simulink model "SWC_ETE_type"  (R2024a)
settings: Solver=FixedStepDiscrete  StartTime=0.0  StopTime=10.0  RelTol=1e-3
values from neighbouring files (symbols this model uses):
  C_FOC_SAMPLE_TIME = single(0.0001)    [vcu_local_hdr.m]
  ENUM_SENSORFOCMODE_CURRENTRDCTEMP = uint8(  2  )    [vcu_local_hdr.m]
  ENUM_SENSORFOCMODE_FAKERDC = uint8(  1  )    [vcu_local_hdr.m]
  ENUM_SENSORFOCMODE_RDCALIGN = uint8(  3  )    [vcu_local_hdr.m]
  ENUM_SENSORMODE_RDC = uint8(  0  )    [vcu_local_hdr.m]
  FALSE = boolean( 0 )    [vcu_local_hdr.m]
  MINUSONE_PI = single( -pi)    [vcu_local_hdr.m]
  PI = single( pi )    [vcu_local_hdr.m]
  SPD_GAIN = single(2*pi/60)    [vcu_local_hdr.m]
  TRUE = boolean( 1 )    [vcu_local_hdr.m]
  TWO_PI = single( 2*pi)    [vcu_local_hdr.m]
  ZERO_FLOAT = single(0)    [vcu_local_hdr.m]
undefined symbols (not defined in the file or in its folder): KFOC_25Amb_degC, KFOC_ADCReadEnum_enum, KFOC_DCBusLPF_c, KFOC_DCBusUseRaw_flg, KFOC_DCBusVoltage_V_ovrdflg, KFOC_DCBusVoltage_V_ovrdval, KFOC_FltActn_flg_ovrdflg, KFOC_FltActn_flg_ovrdfval, KFOC_GateICDisable_flg, KFOC_GateICEnable_flg, KFOC_GateICTempConst_raw, KFOC_IdCmd_A_ovrdflg, KFOC_IdCmd_A_ovrdfval, KFOC_IqCmd_A_ovrdflg, KFOC_IqCmd_A_ovrdfval, KFOC_OpMod_enum, KFOC_OpMod_enum_ovrdflg, KFOC_OpMod_enum_ovrdval, KFOC_PosnOffset_flg_ovrdflg, KFOC_PosnOffset_rad_ovrdval, KFOC_PWMidle_flg, KFOC_RotPosnOffset_rad_ovrdflg, KFOC_RotPosnOffset_rad_ovrdval, KFOC_SensorMode_enum, KFOC_SpdCmd_RPM, KFOC_TCTS_const, KFOC_VdCmd_V, KFOC_VqCmd_V, KFOC_VTS25_V
libraries: simulink x6, rot x2, GRC_Lib x1, pcs_grc x1, rot_grc x1, hdlsllib x1, CCM_FVT x1, dgh_grc x1, pdc_grc x1
(part 1 of 2)
settings Model: DataDictionary=APPTypes.sldd  Creator=FVT22063  LastModifiedBy=FVT22063
settings DataIOCC: SaveFormat=StructureWithTime
settings OptimizationCC: DefaultParameterBehavior=Inlined  EnhancedBackFolding=on  PassReuseOutputArgsAs=Individual arguments  ZeroExternalMemoryAtStartup=off  ZeroInternalMemoryAtStartup=off  OptimizeBlockOrder=speed  DifferentSizesBufferReuse=on  OptimizationCustomize=off  EfficientTunableParamExpr=on
settings DebuggingCC: ParameterTunabilityLossMsg=error
settings HardwareCC: ProdBitPerPointer=32  ProdBitPerSizeT=32  ProdBitPerPtrDiffT=32  ProdLargestAtomicInteger=Long  ProdLargestAtomicFloat=Double  ProdWordSize=32  ProdLongLongMode=on  ProdHWDeviceType=ARM Compatible->ARM Cortex-M
settings ModelReferenceCC: ModelReferenceNumInstancesAllowed=Single
settings SFSimCC: SimCustomHeaderCode="#include \"FVTMC_API.h\""  SimUserSources=FVTMC_API.c  MATLABDynamicMemAlloc=off
settings RTWCC: Description=AUTOSAR  SystemTargetFile=autosar.tlc  GenCodeOnly=on  TemplateMakefile=ert_default_tmf  PortableWordSizes=on
settings CodeAppCC: ForceParamTrailComments=on  IgnoreCustomStorageClasses=off  OperatorAnnotations=on  SimulinkDataObjDesc=on  SFDataObjDesc=on  InsertBlockDesc=on
settings STFCustomTargetCC: UtilityFuncGeneration=Shared location  MultiwordLength=256  ParMdlRefBuildCompliant=on  CompOptLevelCompliant=on  IncludeMdlTerminateFcn=off  CombineOutputUpdateFcns=on  SuppressErrorStatus=on  ERTCustomFileBanners=on  SupportNonFinite=off  SupportComplex=off  SupportContinuousTime=off  SupportNonInlinedSFcns=off  RemoveResetFunc=on  MATLABClassNameForMDSCustomization=Simulink.SoftwareTarget.ERTCustomization  AutosarCompliant=on  GRTInterface=off  GenerateSharedConstants=off  LookupTableObjectStructAxisOrder=2,1,3,4,...  LUTObjectStructOrderEvenSpacing=Size,Table,Breakpoints  SystemTargetFile=autosar.tlc
settings ERTTargetCC: TargetLangStandard=C99 (ISO)  UtilityFuncGeneration=Shared location  ConcurrentExecutionCompliant=off  IncludeMdlTerminateFcn=off  SuppressErrorStatus=on  SupportNonFinite=off  SupportComplex=off  ModelStepFunctionPrototypeControlCompliant=off  CPPClassGenCompliant=off  AutosarCompliant=on  GenerateSharedConstants=off  LookupTableObjectStructAxisOrder=2,1,3,4,...  LUTObjectStructOrderEvenSpacing=Size,Table,Breakpoints  GenerateASAP2=on  InlinedParameterPlacement=NonHierarchical  ERTCustomFileTemplate=example_file_process.tlc  ConvertIfToSwitch=off  SuppressUnreachableDefaultCases=off  BooleanTrueId=true_MatlabRTW  BooleanFalseId=false_MatlabRTW

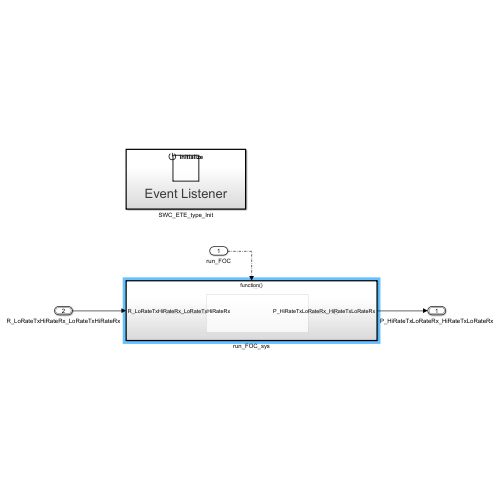
[thumbnail: Simulink's stored preview of the top-level diagram]
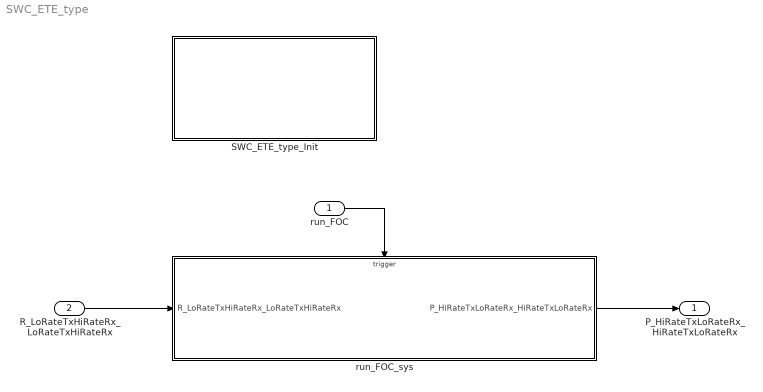
== system SWC_ETE_type ==
  run_FOC : Inport  OutputFunctionCall=on
  R_LoRateTxHiRateRx_LoRateTxHiRateRx : Inport  Port=2  OutDataTypeStr=Bus: DT_LoRateTxHiRateRx  PortDimensions=1  BusOutputAsStruct=on
  SWC_ETE_type_Init : Subsystem
  run_FOC_sys : Subsystem
  P_HiRateTxLoRateRx_HiRateTxLoRateRx : Outport  OutDataTypeStr=Bus: DT_HiRateTxLoRateRx  PortDimensions=1  BusOutputAsStruct=on
  wires:
  R_LoRateTxHiRateRx_LoRateTxHiRateRx/1 -> run_FOC_sys/1(R_LoRateTxHiRateRx_LoRateTxHiRateRx)
  run_FOC_sys/1(P_HiRateTxLoRateRx_HiRateTxLoRateRx) -> P_HiRateTxLoRateRx_HiRateTxLoRateRx/1
  run_FOC/1 -> run_FOC_sys/Trigger

== system SWC_ETE_type/SWC_ETE_type_Init ==
  Event Listener : EventListener  EventName=reset

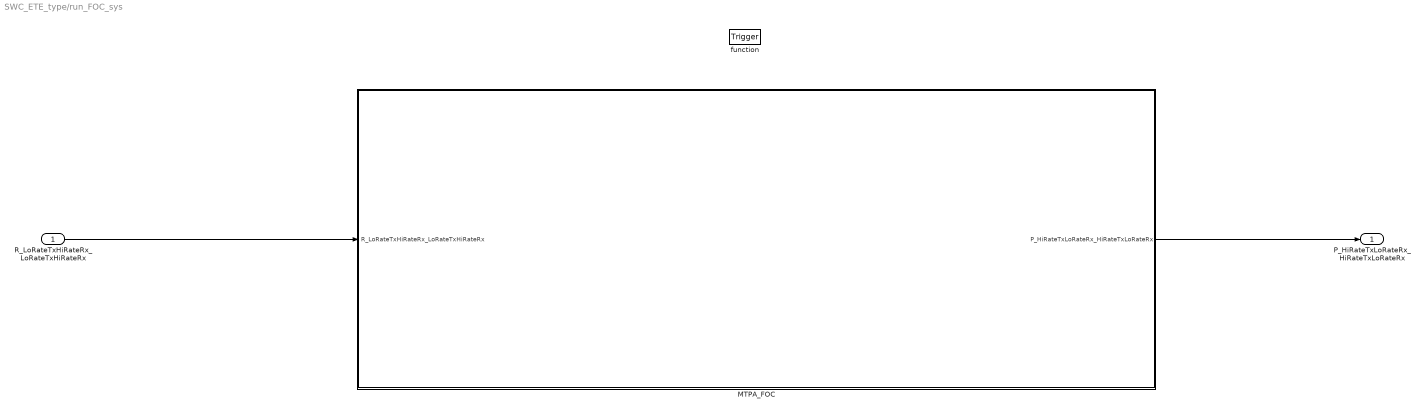
== system SWC_ETE_type/run_FOC_sys ==
  R_LoRateTxHiRateRx_LoRateTxHiRateRx : Inport
  function : TriggerPort  TriggerType=function-call  VariantControl=(inherit)
  MTPA_FOC : Subsystem  TreatAsAtomicUnit=on
      settings: RTWSystemCode=Nonreusable function  RTWFcnNameOpts=Use subsystem name  RTWFileNameOpts=Use subsystem name
  P_HiRateTxLoRateRx_HiRateTxLoRateRx : Outport
  wires:
  R_LoRateTxHiRateRx_LoRateTxHiRateRx/1 -> MTPA_FOC/1(R_LoRateTxHiRateRx_LoRateTxHiRateRx)
  MTPA_FOC/1(P_HiRateTxLoRateRx_HiRateTxLoRateRx) -> P_HiRateTxLoRateRx_HiRateTxLoRateRx/1

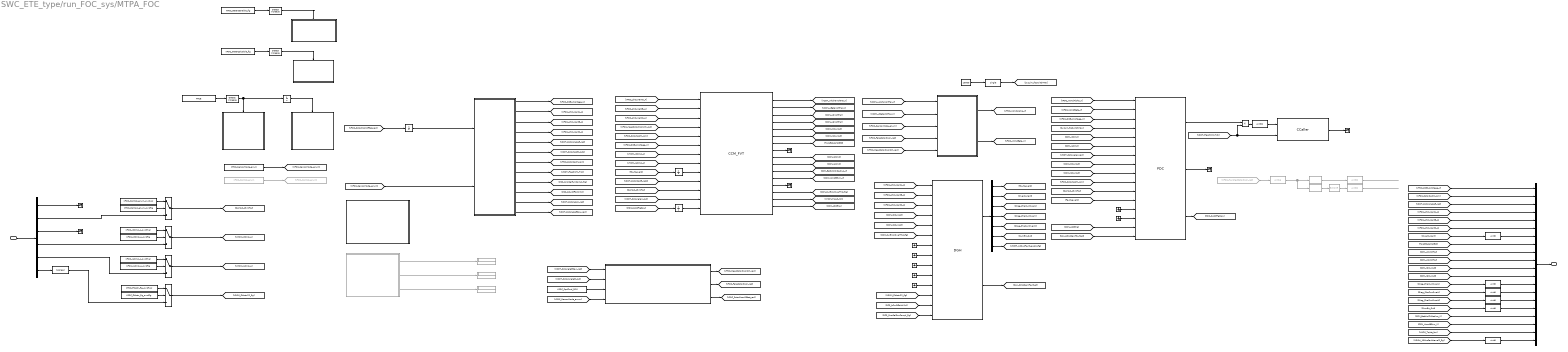
== system SWC_ETE_type/run_FOC_sys/MTPA_FOC ==
  R_LoRateTxHiRateRx_LoRateTxHiRateRx : Inport
  ADC_RDC_Read : Subsystem  TreatAsAtomicUnit=on
      settings: RTWSystemCode=Nonreusable function  RTWFcnNameOpts=Use subsystem name  RTWFileNameOpts=Use subsystem name
  Bit Shift : hdlsllib/Logic and Bit Operations/Bit Shift  Commented=on  mode=Shift Right Logical  N=8
  Bitwise Operator : simulink/Logic and Bit Operations/Bitwise Operator  Commented=on  logicop=AND  UseBitMask=on  BitMask=0xFF00  BitMaskRealWorld=Stored Integer
  Bitwise Operator1 : simulink/Logic and Bit Operations/Bitwise Operator  Commented=on  logicop=AND  UseBitMask=on  BitMask=0x00FF  BitMaskRealWorld=Stored Integer
  Bus Creator : BusCreator  Inputs=20  OutDataTypeStr=Bus: DT_HiRateTxLoRateRx  NonVirtualBus=on
  Bus Selector : BusSelector  OutputSignals=VDGH_FaultLevel2_flg,OverCurrent,Diag_bPhaCurrOverU,Diag_bPhaCurrOverV,Diag_bPhaCurrOverW,SumErr_Out,VDGH_100usFaultLevel2_flg
  Bus Selector1 : BusSelector  OutputSignals=u8_OpMod_stMotAct,u8_OpMod_stIvtrTar,f32_SysLim_frqSwitchMax,f32_VMCM_IdCmd_A,f32_VMCM_IqCmd_A,u8_VDSM_FltActn22_flg
  C Caller1 : CCaller  FunctionName=pwm_set_duty  PortSpecificationStruct="%)30     .      0   8    (     @         %    \"     (    !     0         %  0 \"0    $    _    07)G3F%M90  4&]R=$YA;64 4V-O<&4     26YD97@     5'EP90      4VEZ90      27-';&]B86P   X   !     !@    @    $          4    (     0    X    !         !     .    =3,R07)R87DS7U1I8VL   X   !     !@    @    $          4    (     0    X    !         !     .    =3,R07)R87DS7U1I8VL   X   !     !@    @    $          4    (     0    L    !         !     +    26YP=71/=71P=70       X    X    !@    @    &          4    (     0    $    !          D    (               .    .     8    (    !          %    \"     $    &     0         0    !@   '5I;G0S,@  #@   #     &    \"     0         !0    @    !     0    $         $  ! #,    .    ,     8    (    \"0(        %    \"     $    !     0         \"  $       X   !     !@    @    $          4    (     0    L    !         !     +    <&5R:6]D7U1I8VL       X   !     !@    @    $          4    (     0    L    !         !     +    <&5R:6]D7U1I8VL       X    X    !@    @    $          4    (     0    4    !         !     %    26YP=70    .    .     8    (    !@         %    \"     $    !     0         )    \"            / _#@   #@    &    \"     0         !0    @    !    !@    $         $     8   !U:6YT,S(   X    P    !@    @    $          4    (     0    $    !         !   0 Q    #@   #     &    \"     D\"        !0    @    !     0    $          @ !"
  CCM_FVT : CCM_FVT/CCM_FVT  SystemSampleTime=-1  VariantActivationTime=update diagram  AllowFlexibleInterface=on  Latency=0  AutoFrameSizeCalculation=off
  Cast To Boolean : DataTypeConversion  OutDataTypeStr=boolean  SaturateOnIntegerOverflow=off  RndMeth=Floor
  Constant : Constant  Value=10000
  Constant1 : Constant  Value=KFOC_GateICDisable_flg
  Constant10 : Constant  Value=KFOC_OpMod_enum_ovrdflg
  Constant11 : Constant  Value=KFOC_OpMod_enum_ovrdval
  Constant12 : Constant  Value=KFOC_FltActn_flg_ovrdflg
  Constant13 : Constant  Value=KFOC_SensorMode_enum
  Constant14 : Constant  Value=KFOC_FltActn_flg_ovrdfval
  Constant2 : Constant  Value=KFOC_SpdCmd_RPM
  Constant3 : Constant  Value=KFOC_GateICEnable_flg
  Constant4 : Constant  Commented=on  Value=KFOC_OpMod_enum
  Constant5 : Constant  Value=KFOC_IdCmd_A_ovrdflg
  Constant6 : Constant  Value=KFOC_IdCmd_A_ovrdfval
  Constant7 : Constant  Value=TRUE
  Constant8 : Constant  Value=KFOC_IqCmd_A_ovrdflg
  Constant9 : Constant  Value=KFOC_IqCmd_A_ovrdfval
  DGH : dgh_grc/DGH  SystemSampleTime=-1  VariantActivationTime=update diagram  AllowFlexibleInterface=on  Latency=0  AutoFrameSizeCalculation=off
  Data Type Conversion : DataTypeConversion  OutDataTypeStr=single  SaturateOnIntegerOverflow=off  RndMeth=Floor
  Data Type Conversion1 : DataTypeConversion  OutDataTypeStr=uint32  SaturateOnIntegerOverflow=off  RndMeth=Floor
  Data Type Conversion{2..5,9..10} (6 alike) : DataTypeConversion  OutDataTypeStr=uint8  SaturateOnIntegerOverflow=off  RndMeth=Floor
  Data Type Conversion6 : DataTypeConversion  Commented=on  OutDataTypeStr=uint32  SaturateOnIntegerOverflow=off  RndMeth=Floor
  Data Type Conversion7 : DataTypeConversion  Commented=on  OutDataTypeStr=uint32  SaturateOnIntegerOverflow=off  RndMeth=Floor
  Data Type Conversion8 : DataTypeConversion  Commented=on  OutDataTypeStr=uint16  SaturateOnIntegerOverflow=off  RndMeth=Floor
  Detect Increase : simulink/Logic and Bit Operations/Detect Increase  vinit=0.0  OutDataTypeStr=boolean
  Detect Increase1 : simulink/Logic and Bit Operations/Detect Increase  vinit=0.0  OutDataTypeStr=boolean
  Detect Increase2 : simulink/Logic and Bit Operations/Detect Increase  vinit=0.0  OutDataTypeStr=boolean
  Disable_GateIC : Subsystem
  Display : Display  Commented=on
  Display1 : Display  Commented=on
  Display2 : Display  Commented=on
  Enable_GateIC : Subsystem
  FOC_Mode_Judge : Subsystem  TreatAsAtomicUnit=on
      settings: RTWSystemCode=Nonreusable function  RTWFcnNameOpts=Use subsystem name  RTWFileNameOpts=Use subsystem name
  From42 : From  Commented=on  GotoTag=VFOC_HandledRotorPosn_rad
  GateDirver_Temp_Read : Subsystem  Commented=on  TreatAsAtomicUnit=on
      settings: RTWSystemCode=Nonreusable function  RTWFcnNameOpts=Use subsystem name  RTWFileNameOpts=Use subsystem name
  Goto24 : Goto  Commented=on  GotoTag=VFOC_OpMod_enum
  Ground{,1..6} (7 alike) : Ground
  PDC : pdc_grc/PDC  SystemSampleTime=-1  VariantActivationTime=update diagram  AllowFlexibleInterface=on  Latency=0  AutoFrameSizeCalculation=off
  PWM_idle_Mode : Subsystem
  Product : Product
  RotorPositionHandle : Subsystem
  Subsystem : Subsystem
  Subsystem1 : Subsystem
  Switch{,1..3} (4 alike) : Switch  Criteria=u2 ~= 0  SaturateOnIntegerOverflow=off  InputSameDT=off
  Terminator{,1..5} (6 alike) : Terminator
  Unit Delay{,1..3} (4 alike) : UnitDelay  SampleTime=-1  HasFrameUpgradeWarning=on
  P_HiRateTxLoRateRx_HiRateTxLoRateRx : Outport
  wires:
  Detect Increase/1 -> Unit Delay/1, Subsystem/Enable
  ADC_RDC_Read/1(VFOC_DCBusVoltage_V) -> [VFOC_DCBusVoltage_V]
  Data Type Conversion6/1 -> ?  "RotorPosn_100rad_LowByte"
  [VFOC_SensorMode_enum] -> RotorPositionHandle/4(VFOC_SensorMode_enum)
  RotorPositionHandle/1(VFOC_MeasRotorPosn2Pi_rad) -> [VFOC_MeasRotorPosn2Pi_rad]
  [VCCM_uBetaVoltTar_V] -> FOC_Mode_Judge/2(VCCM_uBetaVoltTar_V)
  Data Type Conversion8/1 -> Bitwise Operator/1, Bitwise Operator1/1
  Constant7/1 -> Detect Increase/1
  ADC_RDC_Read/4(VFOC_phCurrentC_A) -> [VFOC_phCurrentC_A]
  GateDirver_Temp_Read/1(Out1) -> Display/1
  [VFOC_SensorMode_enum] -> FOC_Mode_Judge/3(VFOC_SensorMode_enum)
  Data Type Conversion7/1 -> ?  "RotorPosn_100rad_HighByte"
  [VFOC_MeasRotorPosn2Pi_rad] -> FOC_Mode_Judge/5(VFOC_MeasRotorPosn2Pi_rad)
  [VFOC_FakeRotorPosn_rad] -> FOC_Mode_Judge/4(VFOC_FakeRotorPosn_rad)
  Bit Shift/1 -> Data Type Conversion7/1
  RotorPositionHandle/2(VFOC_FakeRotorPosn_rad) -> [VFOC_FakeRotorPosn_rad]
  Bitwise Operator/1 -> Bit Shift/1
  GateDirver_Temp_Read/2(Out2) -> Display1/1
  ADC_RDC_Read/3(VFOC_phCurrentB_A) -> [VFOC_phCurrentB_A]
  [VFOC_MeasRotorPosn2Pi_rad] -> CCM_FVT/4
  Constant13/1 -> [VFOC_SensorMode_enum]
  GateDirver_Temp_Read/3(Out3) -> Display2/1
  Bitwise Operator1/1 -> Data Type Conversion6/1
  Constant2/1 -> RotorPositionHandle/3(VFOC_SpdCmd_rpm)
  [VCCM_uAlphaVoltTar_V] -> FOC_Mode_Judge/1(VCCM_uAlphaVoltTar_V)
  [VFOC_DCBusVoltage_V] -> CCM_FVT/6
  [VFOC_RotorSpdM_rpm] -> CCM_FVT/5
  ADC_RDC_Read/5(VROT_RotorAngleE_rad) -> [VROT_RotorAngleE_rad]
  [VROT_RotorAngleE_rad] -> RotorPositionHandle/2(VROT_RotorAngleE_rad)
  ADC_RDC_Read/6(VROT_RotorSpdE_rads) -> [VROT_RotorSpdE_rads]
  ADC_RDC_Read/7(VROT_RotorSpdM_rpm) -> [VFOC_RotorSpdM_rpm]
  Unit Delay/1 -> Subsystem1/Enable
  Detect Increase1/1 -> Disable_GateIC/Enable
  Detect Increase2/1 -> Enable_GateIC/Enable
  Constant1/1 -> Detect Increase1/1
  Constant3/1 -> Detect Increase2/1
  FOC_Mode_Judge/1(VFOC_VcmdAlpha_V) -> [VFOC_VcmdAlpha_V]
  FOC_Mode_Judge/2(VFOC_VcmdBeta_V) -> [VFOC_VcmdBeta_V]
  [VFOC_DCBusVoltage_V] -> PDC/3
  [VFOC_RotorSpdM_rpm] -> PDC/10
  ADC_RDC_Read/2(VFOC_phCurrentA_A) -> [VFOC_phCurrentA_A]
  [VFOC_phCurrentA_A] -> CCM_FVT/1
  [VFOC_phCurrentB_A] -> CCM_FVT/2
  [VFOC_phCurrentC_A] -> CCM_FVT/3
  CCM_FVT/1 -> [VCCM_uAlphaVoltTar_V]
  CCM_FVT/2 -> [VCCM_uBetaVoltTar_V]
  CCM_FVT/3 -> [CCM_uDVoltTar]
  CCM_FVT/4 -> [CCM_uQVoltTar]
  [VFOC_VcmdAlpha_V] -> PDC/1
  [VFOC_VcmdBeta_V] -> PDC/2
  [SysLim_frqSwitchMax] -> PDC/4
  Constant/1 -> Data Type Conversion/1
  Data Type Conversion/1 -> [SysLim_frqSwitchMax]
  CCM_FVT/5 -> [CCM_iDCurrAct]
  CCM_FVT/6 -> [CCM_iQCurrAct]
  CCM_FVT/9 -> [CCM_idCmd]
  CCM_FVT/10 -> [CCM_iqCmd]
  [CCM_idCmd] -> PDC/5
  [CCM_iqCmd] -> PDC/6
  [CCM_iDCurrAct] -> PDC/8
  [CCM_iQCurrAct] -> PDC/9
  [VROT_RotorSpdE_rads] -> CCM_FVT/10
  [OpMod_stlvtrTar] -> PDC/11
  [OpMod_stlvtrTar] -> CCM_FVT/11
  Constant4/1 -> Goto24/1
  PDC/1 -> Product/1  "PDC_Ivtr1ModCmd"
  C Caller1/1 -> Terminator/1
  ADC_RDC_Read/8(VROT_FreqPWM_Tick) -> [VROT_FreqPWM_Tick]
  [VROT_FreqPWM_Tick] -> Product/2, C Caller1/2
  CCM_FVT/16 -> [CCM_ASCEna]
  [CCM_ASCEna] -> PDC/15
  Product/1 -> Data Type Conversion1/1
  Data Type Conversion1/1 -> C Caller1/1
  ADC_RDC_Read/11(VROT_RotAngleV_rad) -> [VROT_RotAngleV_rad]
  [VROT_RotAngleV_rad] -> CCM_FVT/12
  [VROT_RotAngleV_rad] -> PDC/7
  PDC/3 -> [PDC_bASCFlgRaw]
  Unit Delay1/1 -> CCM_FVT/13
  [PDC_bASCFlgRaw] -> Unit Delay1/1
  RotorPositionHandle/3(VFOC_RotorPosnOffset_rad) -> [VFOC_RotorPosnOffset_rad]
  [VFOC_RotorPosnOffset_rad] -> Unit Delay2/1
  Unit Delay2/1 -> ADC_RDC_Read/1(VFOC_RotPosnOfstDelay_rad)  "VFOC_RotPosnOfstDelay_rad"
  [CCM_iDCurrAct] -> DGH/4
  [CCM_iQCurrAct] -> DGH/5
  [VFOC_phCurrentA_A] -> DGH/1
  [VFOC_phCurrentC_A] -> DGH/3
  [VFOC_phCurrentB_A] -> DGH/2
  CCM_FVT/14 -> [CCM_CurErrorOverThd_flg]
  [CCM_CurErrorOverThd_flg] -> DGH/6
  [PCS_bCurOffsVolVld] -> DGH/13
  [PCS_SnsrSelfLrnCompl_flg] -> DGH/14
  ADC_RDC_Read/10(PCS_bCurOffsVolVld_flg) -> [PCS_bCurOffsVolVld]
  ADC_RDC_Read/9(PCS_SnsrSelfLrnCompl_flg) -> [PCS_SnsrSelfLrnCompl_flg]
  Unit Delay3/1 -> CCM_FVT/9
  [FaultLevel2] -> Unit Delay3/1
  DGH/2 -> [bsw_bPosSenrFaultLat]
  [bsw_bPosSenrFaultLat] -> PDC/16
  [FaultLevel2] -> PDC/12
  From42/1 -> Data Type Conversion8/1
  DGH/1 -> Bus Selector/1
  Bus Selector/1 -> [FaultLevel2]  "<VDGH_FaultLevel2_flg>"
  R_LoRateTxHiRateRx_LoRateTxHiRateRx/1 -> Bus Selector1/1
  Bus Selector1/1 -> Terminator2/1  "<u8_OpMod_stMotAct>"
  Bus Selector1/2 -> Switch2/3  "<u8_OpMod_stIvtrTar>"
  Bus Selector1/3 -> Terminator1/1  "<f32_SysLim_frqSwitchMax>"
  [VMCM_IdCmd_A] -> CCM_FVT/7
  [VMCM_IqCmd_A] -> CCM_FVT/8
  Bus Selector1/5 -> Switch1/3  "<f32_VMCM_IqCmd_A>"
  [VDSM_FltActn22_flg] -> DGH/12
  Bus Selector1/6 -> Cast To Boolean/1  "<u8_VDSM_FltActn22_flg>"
  Bus Creator/1 -> P_HiRateTxLoRateRx_HiRateTxLoRateRx/1
  [VFOC_DCBusVoltage_V] -> Bus Creator/1
  [VFOC_RotorSpdM_rpm] -> Bus Creator/2
  [VROT_RotorAngleE_rad] -> Bus Creator/3
  [VFOC_phCurrentB_A] -> Bus Creator/5
  [VFOC_phCurrentC_A] -> Bus Creator/6
  [VFOC_phCurrentA_A] -> Bus Creator/4
  Bus Selector/2 -> [OverCurrent]  "<OverCurrent>"
  [OverCurrent] -> Data Type Conversion2/1
  CCM_FVT/7 -> [TorqEst_tqMotEst]
  [TorqEst_tqMotEst] -> Bus Creator/8
  [CCM_uQVoltTar] -> Bus Creator/10
  [CCM_uDVoltTar] -> Bus Creator/9
  [CCM_iDCurrAct] -> Bus Creator/11
  [CCM_iQCurrAct] -> Bus Creator/12
  Bus Selector/3 -> [Diag_PhaCurrOverU]  "<Diag_bPhaCurrOverU>"
  Bus Selector/4 -> [Diag_PhaCurrOverV]  "<Diag_bPhaCurrOverV>"
  Bus Selector/5 -> [Diag_PhaCurrOverW]  "<Diag_bPhaCurrOverW>"
  [Diag_PhaCurrOverU] -> Data Type Conversion3/1
  [Diag_PhaCurrOverV] -> Data Type Conversion4/1
  [Diag_PhaCurrOverW] -> Data Type Conversion5/1
  Bus Selector/6 -> [SumErr_Out]  "<SumErr_Out>"
  [SumErr_Out] -> Data Type Conversion9/1
  CCM_FVT/11 -> [CCM_BattVolCirRadius_V]
  CCM_FVT/12 -> [CCM_VcmdBfLim_V]
  CCM_FVT/15 -> [VMCM_TqAct_Nm]
  [CCM_BattVolCirRadius_V] -> Bus Creator/17
  [CCM_VcmdBfLim_V] -> Bus Creator/18
  [VMCM_TqAct_Nm] -> Bus Creator/19
  Bus Selector/7 -> [VDGH_100usFaultLevel2_flg]  "<VDGH_100usFaultLevel2_flg>"
  [VDGH_100usFaultLevel2_flg] -> Data Type Conversion10/1
  Data Type Conversion2/1 -> Bus Creator/7
  Data Type Conversion3/1 -> Bus Creator/13
  Data Type Conversion4/1 -> Bus Creator/14
  Data Type Conversion5/1 -> Bus Creator/15
  Data Type Conversion9/1 -> Bus Creator/16
  Data Type Conversion10/1 -> Bus Creator/20
  Cast To Boolean/1 -> Switch3/3  "VDSM_FltActn22_flg"
  CCM_FVT/13 -> Terminator3/1
  CCM_FVT/8 -> Terminator4/1
  [VFOC_SensorMode_enum] -> ADC_RDC_Read/2(VFOC_SensorMode_enum)
  PDC/2 -> Terminator5/1
  Ground/1 -> DGH/7
  Ground1/1 -> DGH/8
  Ground2/1 -> DGH/9
  Ground4/1 -> DGH/10
  Ground5/1 -> DGH/11
  Ground3/1 -> PDC/13
  Ground6/1 -> PDC/14
  Switch/1 -> [VMCM_IdCmd_A]
  Bus Selector1/4 -> Switch/3  "<f32_VMCM_IdCmd_A>"
  Constant5/1 -> Switch/2
  Constant6/1 -> Switch/1
  Constant8/1 -> Switch1/2
  Constant9/1 -> Switch1/1
  Switch1/1 -> [VMCM_IqCmd_A]
  Switch2/1 -> [OpMod_stlvtrTar]
  Constant10/1 -> Switch2/2
  Constant11/1 -> Switch2/1
  Switch3/1 -> [VDSM_FltActn22_flg]
  Constant12/1 -> Switch3/2
  Constant14/1 -> Switch3/1
  ADC_RDC_Read/12(VROT_RotAngleERaw_rad) -> [VROT_RotAngleERaw_rad]
  [VROT_RotAngleERaw_rad] -> RotorPositionHandle/1(VROT_RotAngleERaw_rad)

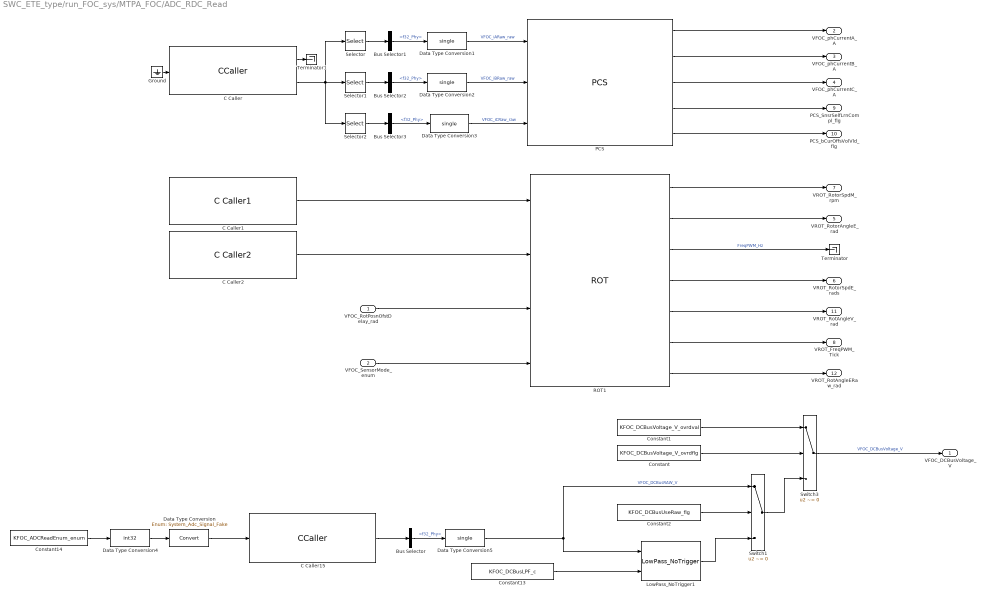
== system SWC_ETE_type/run_FOC_sys/MTPA_FOC/ADC_RDC_Read ==
  VFOC_RotPosnOfstDelay_rad : Inport
  VFOC_SensorMode_enum : Inport  Port=2
  Bus Selector{,1..3} (4 alike) : BusSelector  OutputSignals=f32_Phy
  C Caller : CCaller  FunctionName=read_phase_current_sync_result  PortSpecificationStruct="%)30     .    ^ ,   8    (     @         %    \"     (    !     0         %  0 \"0    $    _    07)G3F%M90  4&]R=$YA;64 4V-O<&4     26YD97@     5'EP90      4VEZ90      27-';&]B86P   X    P    !@    @    $          4    (     0    ,    !         !   P!O=70 #@   #     &    \"     0         !0    @    !     P    $         $  # &]U=  .    .     8    (    !          %    \"     $    &     0         0    !@   $]U='!U=   #@   #@    &    \"     8         !0    @    !     0    $         \"0    @               X    X    !@    @    $          4    (     0    4    !         !     %    =6EN=#@    .    ,     8    (    !          %    \"     $    !     0         0  $ ,0    X    P    !@    @    ) @        4    (     0    $    !          (  0      #@   $     &    \"     0         !0    @    !    \"0    $         $     D   !P:$-U<G)E;G0         #@   $     &    \"     0         !0    @    !    \"0    $         $     D   !P:$-U<G)E;G0         #@   $     &    \"     0         !0    @    !    \"P    $         $     L   !);G!U=$]U='!U=       #@   #@    &    \"     8         !0    @    !     0    $         \"0    @               X   !0    !@    @    $          4    (     0   !X    !         !     >    0G5S.B!%=D%D8U]3:6=N86Q$871A5'EP95]&86ME   .    ,     8    (    !          %    \"     $    !     0         0  $ ,P    X    P    !@    @    ) @        4    (     0    $    !          (  0"
  C Caller1 : rot/ROT/C Caller1  SampleTime=-1
  C Caller15 : CCaller  FunctionName=read_adc_system_value  PortSpecificationStruct="%)30     .    ^ ,   8    (     @         %    \"     (    !     0         %  0 \"0    $    _    07)G3F%M90  4&]R=$YA;64 4V-O<&4     26YD97@     5'EP90      4VEZ90      27-';&]B86P   X    P    !@    @    $          4    (     0    ,    !         !   P!O=70 #@   #     &    \"     0         !0    @    !     P    $         $  # &]U=  .    .     8    (    !          %    \"     $    &     0         0    !@   $]U='!U=   #@   #@    &    \"     8         !0    @    !     0    $         \"0    @               X   !0    !@    @    $          4    (     0   !X    !         !     >    0G5S.B!%=D%D8U]3:6=N86Q$871A5'EP95]&86ME   .    ,     8    (    !          %    \"     $    !     0         0  $ ,0    X    P    !@    @    ) @        4    (     0    $    !          (  0      #@   #@    &    \"     0         !0    @    !    !P    $         $     <   !E4VEG;F%L  X    X    !@    @    $          4    (     0    <    !         !     '    95-I9VYA;  .    .     8    (    !          %    \"     $    %     0         0    !0   $EN<'5T    #@   #@    &    \"     8         !0    @    !     0    $         \"0    @               X   !0    !@    @    $          4    (     0   !P    !         !     <    16YU;3H@4WES=&5M7T%D8U]3:6=N86Q?1F%K90     .    ,     8    (    !          %    \"     $    !     0         0  $ ,0    X    P    !@    @    ) @        4    (     0    $    !          (  0"
  C Caller2 : rot/ROT/C Caller2  SampleTime=-1
  Constant : Constant  Value=KFOC_DCBusVoltage_V_ovrdflg
  Constant1 : Constant  Value=KFOC_DCBusVoltage_V_ovrdval
  Constant13 : Constant  Value=KFOC_DCBusLPF_c
  Constant14 : Constant  Value=KFOC_ADCReadEnum_enum
  Constant2 : Constant  Value=KFOC_DCBusUseRaw_flg
  Data Type Conversion : DataTypeConversion  OutDataTypeStr=Enum: System_Adc_Signal_Fake  SaturateOnIntegerOverflow=off  RndMeth=Floor
  Data Type Conversion{1..3,5} (4 alike) : DataTypeConversion  OutDataTypeStr=single  SaturateOnIntegerOverflow=off  RndMeth=Floor
  Data Type Conversion4 : DataTypeConversion  OutDataTypeStr=int32  SaturateOnIntegerOverflow=off  RndMeth=Floor
  Ground : Ground
  LowPass_NoTrigger1 : GRC_Lib/Filter/LowPass_NoTrigger  IpDT=single
  PCS : pcs_grc/PCS  SystemSampleTime=-1  VariantActivationTime=update diagram  AllowFlexibleInterface=on  Latency=0  AutoFrameSizeCalculation=off
  ROT1 : rot_grc/ROT  SystemSampleTime=-1  VariantActivationTime=update diagram  AllowFlexibleInterface=on  Latency=0  AutoFrameSizeCalculation=off
  Selector : Selector  InputPortWidth=3  IndexOptions=Index vector (dialog)  Indices=1  OutputSizes=1
  Selector1 : Selector  InputPortWidth=3  IndexOptions=Index vector (dialog)  Indices=2  OutputSizes=1
  Selector2 : Selector  InputPortWidth=3  IndexOptions=Index vector (dialog)  Indices=3  OutputSizes=1
  Switch1 : Switch  Criteria=u2 ~= 0  SaturateOnIntegerOverflow=off  InputSameDT=off
      settings: AttributesFormatString=%<Criteria>
  Switch3 : Switch  Criteria=u2 ~= 0  SaturateOnIntegerOverflow=off  InputSameDT=off
      settings: AttributesFormatString=%<Criteria>
  Terminator : Terminator
  Terminator1 : Terminator
  VFOC_DCBusVoltage_V : Outport
  VFOC_phCurrentA_A : Outport  Port=2
  VFOC_phCurrentB_A : Outport  Port=3
  VFOC_phCurrentC_A : Outport  Port=4
  VROT_RotorAngleE_rad : Outport  Port=5
  VROT_RotorSpdE_rads : Outport  Port=6
  VROT_RotorSpdM_rpm : Outport  Port=7
  VROT_FreqPWM_Tick : Outport  Port=8
  PCS_SnsrSelfLrnCompl_flg : Outport  Port=9
  PCS_bCurOffsVolVld_flg : Outport  Port=10
  VROT_RotAngleV_rad : Outport  Port=11
  VROT_RotAngleERaw_rad : Outport  Port=12
  wires:
  Data Type Conversion1/1 -> PCS/1  "VFOC_iARaw_raw"
  Data Type Conversion2/1 -> PCS/2  "VFOC_iBRaw_raw"
  Data Type Conversion3/1 -> PCS/3  "VFOC_iCRaw_raw"
  PCS/3 -> VFOC_phCurrentC_A/1
  PCS/1 -> VFOC_phCurrentA_A/1
  PCS/2 -> VFOC_phCurrentB_A/1
  ROT1/2 -> VROT_RotorAngleE_rad/1
  ROT1/1 -> VROT_RotorSpdM_rpm/1
  ROT1/6 -> VROT_FreqPWM_Tick/1
  ROT1/4 -> VROT_RotorSpdE_rads/1
  LowPass_NoTrigger1/1 -> Switch1/3
  Constant/1 -> Switch3/2
  Constant1/1 -> Switch3/1
  Switch3/1 -> VFOC_DCBusVoltage_V/1  "VFOC_DCBusVoltage_V"
  Constant13/1 -> LowPass_NoTrigger1/2
  Constant14/1 -> Data Type Conversion4/1
  Data Type Conversion4/1 -> Data Type Conversion/1
  C Caller15/1 -> Bus Selector/1
  Data Type Conversion/1 -> C Caller15/1
  Bus Selector/1 -> Data Type Conversion5/1  "<f32_Phy>"
  PCS/4 -> PCS_SnsrSelfLrnCompl_flg/1
  PCS/5 -> PCS_bCurOffsVolVld_flg/1
  C Caller1/1 -> ROT1/1
  C Caller2/1 -> ROT1/2
  ROT1/5 -> VROT_RotAngleV_rad/1
  VFOC_RotPosnOfstDelay_rad/1 -> ROT1/3
  ROT1/3 -> Terminator/1  "FreqPWM_Hz"
  Ground/1 -> C Caller/1
  C Caller/1 -> Terminator1/1
  Selector/1 -> Bus Selector1/1
  Selector1/1 -> Bus Selector2/1
  Selector2/1 -> Bus Selector3/1
  C Caller/2 -> Selector2/1, Selector1/1, Selector/1
  Bus Selector1/1 -> Data Type Conversion1/1  "<f32_Phy>"
  Bus Selector2/1 -> Data Type Conversion2/1  "<f32_Phy>"
  Bus Selector3/1 -> Data Type Conversion3/1  "<f32_Phy>"
  VFOC_SensorMode_enum/1 -> ROT1/4
  Data Type Conversion5/1 -> LowPass_NoTrigger1/1, Switch1/1  "VFOC_DCBusRAW_V"
  Switch1/1 -> Switch3/3
  Constant2/1 -> Switch1/2
  ROT1/7 -> VROT_RotAngleERaw_rad/1

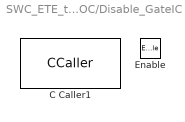
== system SWC_ETE_type/run_FOC_sys/MTPA_FOC/Disable_GateIC ==
  Enable : EnablePort
  C Caller1 : CCaller  FunctionName=gatedriver_disable

== system SWC_ETE_type/run_FOC_sys/MTPA_FOC/Enable_GateIC ==
  Enable : EnablePort
  C Caller : CCaller  FunctionName=gatedriver_enable

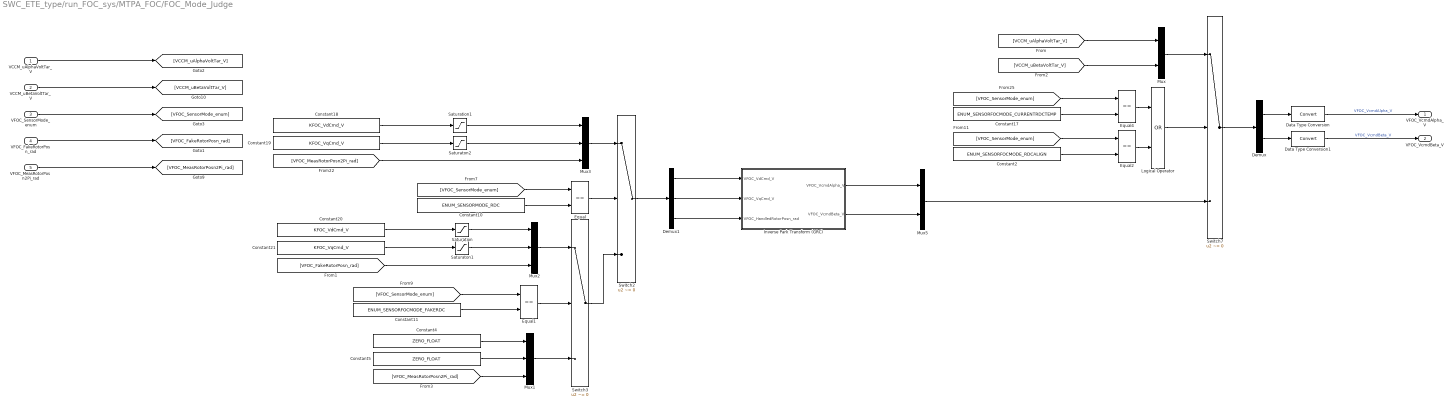
== system SWC_ETE_type/run_FOC_sys/MTPA_FOC/FOC_Mode_Judge ==
  VCCM_uAlphaVoltTar_V : Inport
  VCCM_uBetaVoltTar_V : Inport  Port=2
  VFOC_SensorMode_enum : Inport  Port=3
  VFOC_FakeRotorPosn_rad : Inport  Port=4
  VFOC_MeasRotorPosn2Pi_rad : Inport  Port=5
  Constant10 : Constant  Value=ENUM_SENSORMODE_RDC
  Constant11 : Constant  Value=ENUM_SENSORFOCMODE_FAKERDC
  Constant17 : Constant  Value=ENUM_SENSORFOCMODE_CURRENTRDCTEMP
  Constant18 : Constant  Value=KFOC_VdCmd_V
  Constant19 : Constant  Value=KFOC_VqCmd_V
  Constant2 : Constant  Value=ENUM_SENSORFOCMODE_RDCALIGN
  Constant20 : Constant  Value=KFOC_VdCmd_V
  Constant21 : Constant  Value=KFOC_VqCmd_V
  Constant4 : Constant  Value=ZERO_FLOAT
  Constant5 : Constant  Value=ZERO_FLOAT
  Data Type Conversion : DataTypeConversion  SaturateOnIntegerOverflow=off  RndMeth=Floor
  Data Type Conversion1 : DataTypeConversion  SaturateOnIntegerOverflow=off  RndMeth=Floor
  Demux : Demux  Outputs=2
  Demux1 : Demux  Outputs=3
  Equal{,1..2,4} (4 alike) : RelationalOperator  Operator===  OutDataTypeStr=boolean  RndMeth=Simplest  InputSameDT=off
  Inverse Park Transform (GRC) : Subsystem
  Logical Operator : Logic  Operator=OR  AllPortsSameDT=off  OutDataTypeStr=boolean
  Mux : Mux  Inputs=2
  Mux1 : Mux  Inputs=3
  Mux2 : Mux  Inputs=3
  Mux3 : Mux  Inputs=3
  Mux5 : Mux  Inputs=2
  Saturation : Saturate  UpperLimit=57  LowerLimit=-57
      settings: AttributesFormatString=|
      | Uppder bound: %<UpperLimit>
      | Lower bound: %<LowerLimit>
  Saturation1 : Saturate  UpperLimit=57  LowerLimit=-57
      settings: AttributesFormatString=|
      | Uppder bound: %<UpperLimit>
      | Lower bound: %<LowerLimit>
  Saturaton1 : Saturate  UpperLimit=57  LowerLimit=-57
      settings: AttributesFormatString=|
      | Uppder bound: %<UpperLimit>
      | Lower bound: %<LowerLimit>
  Saturaton2 : Saturate  UpperLimit=57  LowerLimit=-57
      settings: AttributesFormatString=|
      | Uppder bound: %<UpperLimit>
      | Lower bound: %<LowerLimit>
  Switch2 : Switch  Criteria=u2 ~= 0  SaturateOnIntegerOverflow=off  InputSameDT=off
      settings: AttributesFormatString=%<Criteria>
  Switch3 : Switch  Criteria=u2 ~= 0  SaturateOnIntegerOverflow=off  InputSameDT=off
      settings: AttributesFormatString=%<Criteria>
  Switch7 : Switch  Criteria=u2 ~= 0  SaturateOnIntegerOverflow=off  InputSameDT=off
      settings: AttributesFormatString=%<Criteria>
  VFOC_VcmdAlpha_V : Outport
  VFOC_VcmdBeta_V : Outport  Port=2
  wires:
  Constant10/1 -> Equal/2
  Switch3/1 -> Switch2/3
  Equal/1 -> Switch2/2
  Constant11/1 -> Equal1/2
  [VFOC_SensorMode_enum] -> Equal1/1
  Equal1/1 -> Switch3/2
  Demux/1 -> Data Type Conversion/1
  Demux/2 -> Data Type Conversion1/1
  VCCM_uAlphaVoltTar_V/1 -> [VCCM_uAlphaVoltTar_V]
  VCCM_uBetaVoltTar_V/1 -> [VCCM_uBetaVoltTar_V]
  [VCCM_uAlphaVoltTar_V] -> Mux/1
  [VCCM_uBetaVoltTar_V] -> Mux/2
  [VFOC_FakeRotorPosn_rad] -> Mux2/3
  Mux2/1 -> Switch3/1
  Data Type Conversion/1 -> VFOC_VcmdAlpha_V/1  "VFOC_VcmdAlpha_V"
  Data Type Conversion1/1 -> VFOC_VcmdBeta_V/1  "VFOC_VcmdBeta_V"
  [VFOC_SensorMode_enum] -> Equal/1
  Switch7/1 -> Demux/1
  Constant17/1 -> Equal4/2
  [VFOC_SensorMode_enum] -> Equal4/1
  Equal4/1 -> Logical Operator/1
  Mux/1 -> Switch7/1
  Constant19/1 -> Saturaton2/1
  Constant18/1 -> Saturation1/1
  [VFOC_MeasRotorPosn2Pi_rad] -> Mux3/3
  Mux3/1 -> Switch2/1
  Constant20/1 -> Saturation/1
  Constant21/1 -> Saturaton1/1
  Saturation/1 -> Mux2/1
  Saturaton1/1 -> Mux2/2
  Saturation1/1 -> Mux3/1
  Saturaton2/1 -> Mux3/2
  VFOC_SensorMode_enum/1 -> [VFOC_SensorMode_enum]
  VFOC_FakeRotorPosn_rad/1 -> [VFOC_FakeRotorPosn_rad]
  VFOC_MeasRotorPosn2Pi_rad/1 -> [VFOC_MeasRotorPosn2Pi_rad]
  Switch2/1 -> Demux1/1
  Demux1/1 -> Inverse Park Transform (GRC)/1(VFOC_VdCmd_V)
  Demux1/2 -> Inverse Park Transform (GRC)/2(VFOC_VqCmd_V)
  Demux1/3 -> Inverse Park Transform (GRC)/3(VFOC_HandledRotorPosn_rad)
  Inverse Park Transform (GRC)/1(VFOC_VcmdAlpha_V) -> Mux5/1
  Inverse Park Transform (GRC)/2(VFOC_VcmdBeta_V) -> Mux5/2
  Mux5/1 -> Switch7/3
  Constant2/1 -> Equal2/2
  Equal2/1 -> Logical Operator/2
  [VFOC_SensorMode_enum] -> Equal2/1
  Mux1/1 -> Switch3/3
  Constant4/1 -> Mux1/1
  Constant5/1 -> Mux1/2
  [VFOC_MeasRotorPosn2Pi_rad] -> Mux1/3
  Logical Operator/1 -> Switch7/2

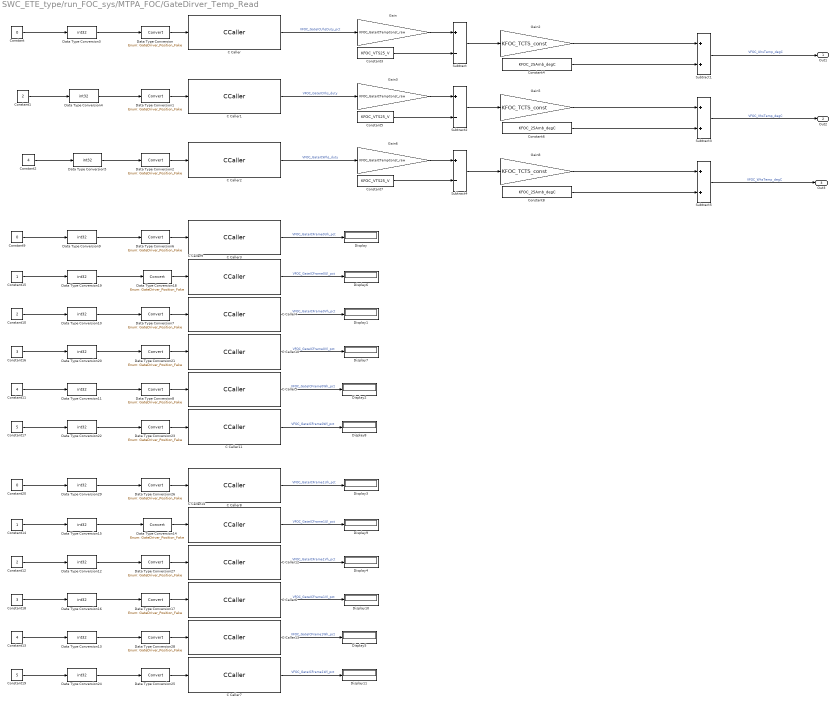
== system SWC_ETE_type/run_FOC_sys/MTPA_FOC/GateDirver_Temp_Read ==
  C Caller : CCaller  FunctionName=get_gatedriver_data_adc  PortSpecificationStruct="%)30     .    X ,   8    (     @         %    \"     (    !     0         %  0 \"0    $    _    07)G3F%M90  4&]R=$YA;64 4V-O<&4     26YD97@     5'EP90      4VEZ90      27-';&]B86P   X    P    !@    @    $          4    (     0    ,    !         !   P!O=70 #@   #     &    \"     0         !0    @    !     P    $         $  # &]U=  .    .     8    (    !          %    \"     $    &     0         0    !@   $]U='!U=   #@   #@    &    \"     8         !0    @    !     0    $         \"0    @               X    X    !@    @    $          4    (     0    8    !         !     &    <VEN9VQE   .    ,     8    (    !          %    \"     $    !     0         0  $ ,0    X    P    !@    @    ) @        4    (     0    $    !          (  0      #@   #@    &    \"     0         !0    @    !    \"     $         $     @   !P;W-I=&EO;@X    X    !@    @    $          4    (     0    @    !         !     (    <&]S:71I;VX.    .     8    (    !          %    \"     $    %     0         0    !0   $EN<'5T    #@   #@    &    \"     8         !0    @    !     0    $         \"0    @               X   !0    !@    @    $          4    (     0   !X    !         !     >    16YU;3H@1V%T941R:79E<E]0;W-I=&EO;E]&86ME   .    ,     8    (    !          %    \"     $    !     0         0  $ ,0    X    P    !@    @    ) @        4    (     0    $    !          (  0"
  C Caller1 : CCaller  FunctionName=get_gatedriver_data_adc  PortSpecificationStruct="%)30     .    X ,   8    (     @         %    \"     (    !     0         %  0 \"0    $    _    07)G3F%M90  4&]R=$YA;64 4V-O<&4     26YD97@     5'EP90      4VEZ90      27-';&]B86P   X    P    !@    @    $          4    (     0    ,    !         !   P!O=70 #@   #     &    \"     0         !0    @    !     P    $         $  # &]U=  .    .     8    (    !          %    \"     $    &     0         0    !@   $]U='!U=   #@   #@    &    \"     8         !0    @    !     0    $         \"0    @               X    X    !@    @    $          4    (     0    8    !         !     &    <VEN9VQE   .    ,     8    (    !          %    \"     $    !     0         0  $ ,0    X    P    !@    @    ) @        4    (     0    $    !          (  0      #@   #@    &    \"     0         !0    @    !    \"     $         $     @   !P;W-I=&EO;@X    X    !@    @    $          4    (     0    @    !         !     (    <&]S:71I;VX.    .     8    (    !          %    \"     $    %     0         0    !0   $EN<'5T    #@   #@    &    \"     8         !0    @    !     0    $         \"0    @               X   !0    !@    @    $          4    (     0   !X    !         !     >    16YU;3H@1V%T941R:79E<E]0;W-I=&EO;E]&86ME   .    ,     8    (    !          %    \"     $    !     0         0  $ ,0    X    P    !@    @    ) @        4    (     0    $    !          (  0"
  C Caller{3..5,9..11} (6 alike) : CCaller  FunctionName=get_gatedriver_data_diagnostic1  PortSpecificationStruct="%)30     .    X ,   8    (     @         %    \"     (    !     0         %  0 \"0    $    _    07)G3F%M90  4&]R=$YA;64 4V-O<&4     26YD97@     5'EP90      4VEZ90      27-';&]B86P   X    P    !@    @    $          4    (     0    ,    !         !   P!O=70 #@   #     &    \"     0         !0    @    !     P    $         $  # &]U=  .    .     8    (    !          %    \"     $    &     0         0    !@   $]U='!U=   #@   #@    &    \"     8         !0    @    !     0    $         \"0    @               X    X    !@    @    $          4    (     0    8    !         !     &    <VEN9VQE   .    ,     8    (    !          %    \"     $    !     0         0  $ ,0    X    P    !@    @    ) @        4    (     0    $    !          (  0      #@   #@    &    \"     0         !0    @    !    \"     $         $     @   !P;W-I=&EO;@X    X    !@    @    $          4    (     0    @    !         !     (    <&]S:71I;VX.    .     8    (    !          %    \"     $    %     0         0    !0   $EN<'5T    #@   #@    &    \"     8         !0    @    !     0    $         \"0    @               X   !0    !@    @    $          4    (     0   !X    !         !     >    16YU;3H@1V%T941R:79E<E]0;W-I=&EO;E]&86ME   .    ,     8    (    !          %    \"     $    !     0         0  $ ,0    X    P    !@    @    ) @        4    (     0    $    !          (  0"
  C Caller{6..8,12..14} (6 alike) : CCaller  FunctionName=get_gatedriver_data_diagnostic2  PortSpecificationStruct="%)30     .    X ,   8    (     @         %    \"     (    !     0         %  0 \"0    $    _    07)G3F%M90  4&]R=$YA;64 4V-O<&4     26YD97@     5'EP90      4VEZ90      27-';&]B86P   X    P    !@    @    $          4    (     0    ,    !         !   P!O=70 #@   #     &    \"     0         !0    @    !     P    $         $  # &]U=  .    .     8    (    !          %    \"     $    &     0         0    !@   $]U='!U=   #@   #@    &    \"     8         !0    @    !     0    $         \"0    @               X    X    !@    @    $          4    (     0    8    !         !     &    <VEN9VQE   .    ,     8    (    !          %    \"     $    !     0         0  $ ,0    X    P    !@    @    ) @        4    (     0    $    !          (  0      #@   #@    &    \"     0         !0    @    !    \"     $         $     @   !P;W-I=&EO;@X    X    !@    @    $          4    (     0    @    !         !     (    <&]S:71I;VX.    .     8    (    !          %    \"     $    %     0         0    !0   $EN<'5T    #@   #@    &    \"     8         !0    @    !     0    $         \"0    @               X   !0    !@    @    $          4    (     0   !X    !         !     >    16YU;3H@1V%T941R:79E<E]0;W-I=&EO;E]&86ME   .    ,     8    (    !          %    \"     $    !     0         0  $ ,0    X    P    !@    @    ) @        4    (     0    $    !          (  0"
  C Caller2 : CCaller  FunctionName=get_gatedriver_data_adc  PortSpecificationStruct="%)30     .    X ,   8    (     @         %    \"     (    !     0         %  0 \"0    $    _    07)G3F%M90  4&]R=$YA;64 4V-O<&4     26YD97@     5'EP90      4VEZ90      27-';&]B86P   X    P    !@    @    $          4    (     0    ,    !         !   P!O=70 #@   #     &    \"     0         !0    @    !     P    $         $  # &]U=  .    .     8    (    !          %    \"     $    &     0         0    !@   $]U='!U=   #@   #@    &    \"     8         !0    @    !     0    $         \"0    @               X    X    !@    @    $          4    (     0    8    !         !     &    <VEN9VQE   .    ,     8    (    !          %    \"     $    !     0         0  $ ,0    X    P    !@    @    ) @        4    (     0    $    !          (  0      #@   #@    &    \"     0         !0    @    !    \"     $         $     @   !P;W-I=&EO;@X    X    !@    @    $          4    (     0    @    !         !     (    <&]S:71I;VX.    .     8    (    !          %    \"     $    %     0         0    !0   $EN<'5T    #@   #@    &    \"     8         !0    @    !     0    $         \"0    @               X   !0    !@    @    $          4    (     0   !X    !         !     >    16YU;3H@1V%T941R:79E<E]0;W-I=&EO;E]&86ME   .    ,     8    (    !          %    \"     $    !     0         0  $ ,0    X    P    !@    @    ) @        4    (     0    $    !          (  0"
  Constant : Constant  Value=0
  Constant1 : Constant  Value=2
  Constant10 : Constant  Value=2
  Constant11 : Constant  Value=4
  Constant12 : Constant  Value=2
  Constant13 : Constant  Value=4
  Constant14 : Constant
  Constant15 : Constant
  Constant16 : Constant  Value=3
  Constant17 : Constant  Value=5
  Constant18 : Constant  Value=3
  Constant19 : Constant  Value=5
  Constant2 : Constant  Value=4
  Constant20 : Constant  Value=0
  Constant3 : Constant  Value=KFOC_VTS25_V
  Constant4 : Constant  Value=KFOC_25Amb_degC
  Constant5 : Constant  Value=KFOC_VTS25_V
  Constant6 : Constant  Value=KFOC_25Amb_degC
  Constant7 : Constant  Value=KFOC_VTS25_V
  Constant8 : Constant  Value=KFOC_25Amb_degC
  Constant9 : Constant  Value=0
  Data Type Conversion{,1..2,6..8,14,17..18,21,23,26..28} (14 alike) : DataTypeConversion  OutDataTypeStr=Enum: GateDriver_Position_Fake  SaturateOnIntegerOverflow=off  RndMeth=Floor
  Data Type Conversion{3..5,9..13,15..16,19..20,22,24,29} (15 alike) : DataTypeConversion  OutDataTypeStr=int32  SaturateOnIntegerOverflow=off  RndMeth=Floor
  Data Type Conversion25 : DataTypeConversion  SaturateOnIntegerOverflow=off  RndMeth=Floor
  Display{,1..11} (12 alike) : Display
  Gain : Gain  Gain=KFOC_GateICTempConst_raw
  Gain2 : Gain  Gain=KFOC_TCTS_const
  Gain3 : Gain  Gain=KFOC_GateICTempConst_raw
  Gain5 : Gain  Gain=KFOC_TCTS_const
  Gain6 : Gain  Gain=KFOC_GateICTempConst_raw
  Gain8 : Gain  Gain=KFOC_TCTS_const
  Subtract : Sum  Inputs=+-
  Subtract1 : Sum
  Subtract2 : Sum  Inputs=+-
  Subtract3 : Sum
  Subtract4 : Sum  Inputs=+-
  Subtract5 : Sum
  Out1 : Outport
  Out2 : Outport  Port=2
  Out3 : Outport  Port=3
  wires:
  C Caller/1 -> Gain/1  "VFOC_GateICUhsDuty_pct"
  Constant1/1 -> Data Type Conversion4/1
  Data Type Conversion/1 -> C Caller/1
  Data Type Conversion1/1 -> C Caller1/1
  Constant2/1 -> Data Type Conversion5/1
  Data Type Conversion2/1 -> C Caller2/1
  Gain/1 -> Subtract/1
  Constant3/1 -> Subtract/2
  Gain2/1 -> Subtract1/1
  Subtract1/1 -> Out1/1  "VFOC_UhsTemp_degC"
  Subtract/1 -> Gain2/1
  Constant4/1 -> Subtract1/2
  Constant/1 -> Data Type Conversion3/1
  Constant5/1 -> Subtract2/2
  C Caller1/1 -> Gain3/1  "VFOC_GateICVhs_duty"
  Subtract3/1 -> Out2/1  "VFOC_VhsTemp_degC"
  Gain3/1 -> Subtract2/1
  Subtract2/1 -> Gain5/1
  Gain5/1 -> Subtract3/1
  Constant6/1 -> Subtract3/2
  Constant7/1 -> Subtract4/2
  Gain6/1 -> Subtract4/1
  Gain8/1 -> Subtract5/1
  Subtract4/1 -> Gain8/1
  Subtract5/1 -> Out3/1  "VFOC_WhsTemp_degC"
  C Caller2/1 -> Gain6/1  "VFOC_GateICWhs_duty"
  Constant8/1 -> Subtract5/2
  Data Type Conversion3/1 -> Data Type Conversion/1
  Data Type Conversion4/1 -> Data Type Conversion1/1
  Data Type Conversion5/1 -> Data Type Conversion2/1
  Data Type Conversion11/1 -> Data Type Conversion8/1
  Constant10/1 -> Data Type Conversion10/1
  Data Type Conversion8/1 -> C Caller5/1
  Data Type Conversion9/1 -> Data Type Conversion6/1
  Data Type Conversion10/1 -> Data Type Conversion7/1
  Data Type Conversion6/1 -> C Caller3/1
  Constant9/1 -> Data Type Conversion9/1
  Data Type Conversion7/1 -> C Caller4/1
  Constant11/1 -> Data Type Conversion11/1
  C Caller3/1 -> Display/1  "VFOC_GateICFrame0Uh_pct"
  C Caller4/1 -> Display1/1  "VFOC_GateICFrame0Vh_pct"
  C Caller5/1 -> Display2/1  "VFOC_GateICFrame0Wh_pct"
  C Caller9/1 -> Display6/1  "VFOC_GateICFrame0Ul_pct"
  Data Type Conversion18/1 -> C Caller9/1
  Constant15/1 -> Data Type Conversion19/1
  Data Type Conversion19/1 -> Data Type Conversion18/1
  Constant16/1 -> Data Type Conversion20/1
  C Caller10/1 -> Display7/1  "VFOC_GateICFrame0Vl_pct"
  Data Type Conversion21/1 -> C Caller10/1
  Data Type Conversion20/1 -> Data Type Conversion21/1
  C Caller11/1 -> Display8/1  "VFOC_GateICFrame0Wl_pct"
  Constant17/1 -> Data Type Conversion22/1
  Data Type Conversion23/1 -> C Caller11/1
  Data Type Conversion22/1 -> Data Type Conversion23/1
  C Caller14/1 -> Display9/1  "VFOC_GateICFrame1Ul_pct"
  Data Type Conversion24/1 -> Data Type Conversion25/1
  Data Type Conversion25/1 -> C Caller7/1
  C Caller13/1 -> Display5/1  "VFOC_GateICFrame1Wh_pct"
  C Caller6/1 -> Display10/1  "VFOC_GateICFrame1Vl_pct"
  Data Type Conversion16/1 -> Data Type Conversion17/1
  Data Type Conversion14/1 -> C Caller14/1
  C Caller12/1 -> Display4/1  "VFOC_GateICFrame1Vh_pct"
  Data Type Conversion26/1 -> C Caller8/1
  Constant12/1 -> Data Type Conversion12/1
  Data Type Conversion13/1 -> Data Type Conversion28/1
  Data Type Conversion27/1 -> C Caller12/1
  Constant19/1 -> Data Type Conversion24/1
  Constant14/1 -> Data Type Conversion15/1
  Constant13/1 -> Data Type Conversion13/1
  Constant18/1 -> Data Type Conversion16/1
  Data Type Conversion12/1 -> Data Type Conversion27/1
  Constant20/1 -> Data Type Conversion29/1
  Data Type Conversion29/1 -> Data Type Conversion26/1
  C Caller7/1 -> Display11/1  "VFOC_GateICFrame1Wl_pct"
  Data Type Conversion17/1 -> C Caller6/1
  Data Type Conversion28/1 -> C Caller13/1
  C Caller8/1 -> Display3/1  "VFOC_GateICFrame1Uh_pct"
  Data Type Conversion15/1 -> Data Type Conversion14/1

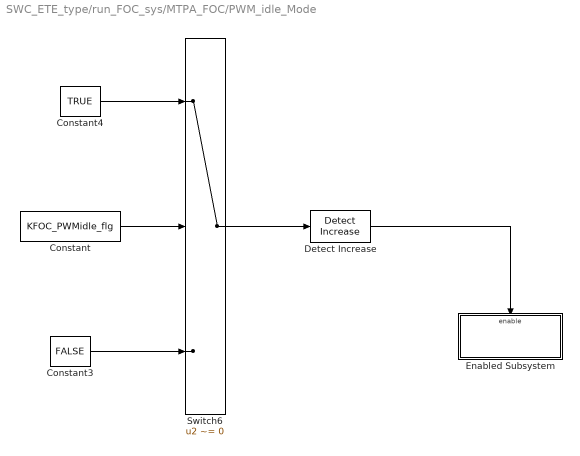
== system SWC_ETE_type/run_FOC_sys/MTPA_FOC/PWM_idle_Mode ==
  Constant : Constant  Value=KFOC_PWMidle_flg
  Constant3 : Constant  Value=FALSE
  Constant4 : Constant  Value=TRUE
  Detect Increase : simulink/Logic and Bit Operations/Detect Increase  vinit=0.0  OutDataTypeStr=boolean
  Enabled Subsystem : Subsystem  TreatAsAtomicUnit=on
  Switch6 : Switch  Criteria=u2 ~= 0  SaturateOnIntegerOverflow=off  InputSameDT=off
      settings: AttributesFormatString=%<Criteria>
  wires:
  Constant4/1 -> Switch6/1
  Constant/1 -> Switch6/2
  Constant3/1 -> Switch6/3
  Switch6/1 -> Detect Increase/1
  Detect Increase/1 -> Enabled Subsystem/Enable

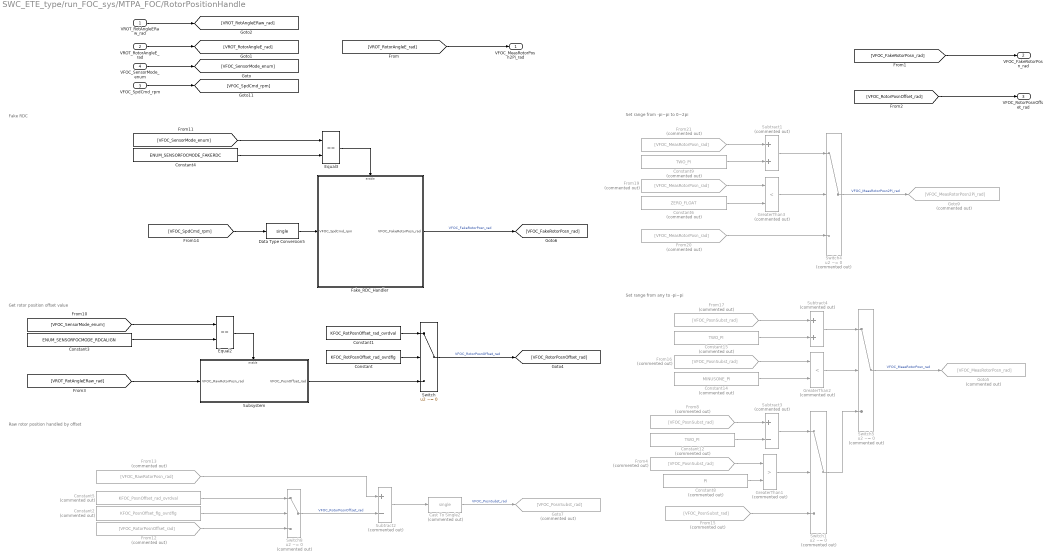
== system SWC_ETE_type/run_FOC_sys/MTPA_FOC/RotorPositionHandle ==
  note: Set range from -pi~pi to 0~2pi
  note: Fake RDC
  note: Get rotor position offset value
  note: Raw rotor position handled by offset
  note: Set range from any to -pi~pi
  VROT_RotAngleERaw_rad : Inport
  VROT_RotorAngleE_rad : Inport  Port=2
  VFOC_SpdCmd_rpm : Inport  Port=3
  VFOC_SensorMode_enum : Inport  Port=4
  Cast To Single2 : DataTypeConversion  Commented=on  OutDataTypeStr=single  SaturateOnIntegerOverflow=off  RndMeth=Floor
  Constant : Constant  Value=KFOC_RotPosnOffset_rad_ovrdflg
  Constant1 : Constant  Value=KFOC_RotPosnOffset_rad_ovrdval
  Constant12 : Constant  Commented=on  Value=TWO_PI
  Constant14 : Constant  Commented=on  Value=MINUSONE_PI
  Constant15 : Constant  Commented=on  Value=TWO_PI
  Constant2 : Constant  Commented=on  Value=KFOC_PosnOffset_flg_ovrdflg
  Constant3 : Constant  Value=ENUM_SENSORFOCMODE_RDCALIGN
  Constant4 : Constant  Value=ENUM_SENSORFOCMODE_FAKERDC
  Constant5 : Constant  Commented=on  Value=KFOC_PosnOffset_rad_ovrdval
  Constant6 : Constant  Commented=on  Value=ZERO_FLOAT
  Constant8 : Constant  Commented=on  Value=PI
  Constant9 : Constant  Commented=on  Value=TWO_PI
  Data Type Conversion5 : DataTypeConversion  OutDataTypeStr=single  SaturateOnIntegerOverflow=off  RndMeth=Floor
  Equal2 : RelationalOperator  Operator===  OutDataTypeStr=boolean  RndMeth=Simplest  InputSameDT=off
  Equal3 : RelationalOperator  Operator===  OutDataTypeStr=boolean  RndMeth=Simplest  InputSameDT=off
  Fake_RDC_Handler : Subsystem  TreatAsAtomicUnit=on
      settings: RTWSystemCode=Nonreusable function  RTWFcnNameOpts=Use subsystem name  RTWFileNameOpts=Use subsystem name
  From12 : From  Commented=on  GotoTag=VFOC_RotorPosnOffset_rad
  From13 : From  Commented=on  GotoTag=VFOC_RawRotorPosn_rad
  From{4,8,15..17} (5 alike) : From  Commented=on  GotoTag=VFOC_PosnSubst_rad
  From19 : From  Commented=on  GotoTag=VFOC_MeasRotorPosn_rad
  From20 : From  Commented=on  GotoTag=VFOC_MeasRotorPosn_rad
  From21 : From  Commented=on  GotoTag=VFOC_MeasRotorPosn_rad
  Goto5 : Goto  Commented=on  GotoTag=VFOC_MeasRotorPosn_rad
  Goto7 : Goto  Commented=on  GotoTag=VFOC_PosnSubst_rad
  Goto9 : Goto  Commented=on  GotoTag=VFOC_MeasRotorPosn2Pi_rad
  GreaterThan1 : RelationalOperator  Commented=on  Operator=>  OutDataTypeStr=boolean  RndMeth=Simplest  InputSameDT=off
  GreaterThan2 : RelationalOperator  Commented=on  Operator=<  OutDataTypeStr=boolean  RndMeth=Simplest  InputSameDT=off
  GreaterThan3 : RelationalOperator  Commented=on  Operator=<  OutDataTypeStr=boolean  RndMeth=Simplest  InputSameDT=off
  Subsystem : Subsystem
  Subtract1 : Sum  Commented=on
  Subtract2 : Sum  Commented=on  Inputs=+-
  Subtract3 : Sum  Commented=on  Inputs=+-
  Subtract4 : Sum  Commented=on
  Switch : Switch  Criteria=u2 ~= 0  SaturateOnIntegerOverflow=off  InputSameDT=off
  Switch{1,4..5,8} (4 alike) : Switch  Commented=on  Criteria=u2 ~= 0  SaturateOnIntegerOverflow=off  InputSameDT=off
      settings: AttributesFormatString=%<Criteria>
  VFOC_MeasRotorPosn2Pi_rad : Outport
  VFOC_FakeRotorPosn_rad : Outport  Port=2
  VFOC_RotorPosnOffset_rad : Outport  Port=3
  wires:
  Constant5/1 -> Switch8/1
  Constant9/1 -> Subtract1/2
  Constant12/1 -> Subtract3/2
  [VFOC_SensorMode_enum] -> Equal3/1
  From16/1 -> GreaterThan2/1
  Subtract1/1 -> Switch4/1
  Switch4/1 -> Goto9/1  "VFOC_MeasRotorPosn2Pi_rad"
  Equal3/1 -> Fake_RDC_Handler/Enable
  From12/1 -> Switch8/3
  Data Type Conversion5/1 -> Fake_RDC_Handler/1(VFOC_SpdCmd_rpm)
  [VFOC_SpdCmd_rpm] -> Data Type Conversion5/1
  GreaterThan2/1 -> Switch5/2
  From15/1 -> Switch1/3
  Subtract4/1 -> Switch5/1
  Fake_RDC_Handler/1(VFOC_FakeRotorPosn_rad) -> [VFOC_FakeRotorPosn_rad]  "VFOC_FakeRotorPosn_rad"
  Constant15/1 -> Subtract4/2
  Constant2/1 -> Switch8/2
  From4/1 -> GreaterThan1/1
  From8/1 -> Subtract3/1
  Cast To Single2/1 -> Goto7/1  "VFOC_PosnSubst_rad"
  Constant4/1 -> Equal3/2
  GreaterThan3/1 -> Switch4/2
  From13/1 -> Subtract2/1
  From21/1 -> Subtract1/1
  From20/1 -> Switch4/3
  Switch1/1 -> Switch5/3
  Constant8/1 -> GreaterThan1/2
  Constant6/1 -> GreaterThan3/2
  From19/1 -> GreaterThan3/1
  Constant14/1 -> GreaterThan2/2
  Subtract3/1 -> Switch1/1
  GreaterThan1/1 -> Switch1/2
  From17/1 -> Subtract4/1
  Subtract2/1 -> Cast To Single2/1
  Equal2/1 -> Subsystem/Enable
  [VFOC_SensorMode_enum] -> Equal2/1
  Switch5/1 -> Goto5/1  "VFOC_MeasRotorPosn_rad"
  [VROT_RotAngleERaw_rad] -> Subsystem/1(VFOC_RawRotorPosn_rad)
  Constant3/1 -> Equal2/2
  Switch8/1 -> Subtract2/2  "VFOC_RotorPosnOffset_rad"
  VFOC_SensorMode_enum/1 -> [VFOC_SensorMode_enum]
  [VROT_RotorAngleE_rad] -> VFOC_MeasRotorPosn2Pi_rad/1
  [VFOC_FakeRotorPosn_rad] -> VFOC_FakeRotorPosn_rad/1
  VROT_RotorAngleE_rad/1 -> [VROT_RotorAngleE_rad]
  VFOC_SpdCmd_rpm/1 -> [VFOC_SpdCmd_rpm]
  Subsystem/1(VFOC_PosnOffset_rad) -> Switch/3
  [VFOC_RotorPosnOffset_rad] -> VFOC_RotorPosnOffset_rad/1
  Switch/1 -> [VFOC_RotorPosnOffset_rad]  "VFOC_RotorPosnOffset_rad"
  Constant/1 -> Switch/2
  Constant1/1 -> Switch/1
  VROT_RotAngleERaw_rad/1 -> [VROT_RotAngleERaw_rad]

== system SWC_ETE_type/run_FOC_sys/MTPA_FOC/Subsystem ==
  Enable : EnablePort
  C Caller : CCaller  FunctionName=Ifx_SvmF32_init

== system SWC_ETE_type/run_FOC_sys/MTPA_FOC/Subsystem1 ==
  Enable : EnablePort
  C Caller : CCaller  FunctionName=gatedriver_enable

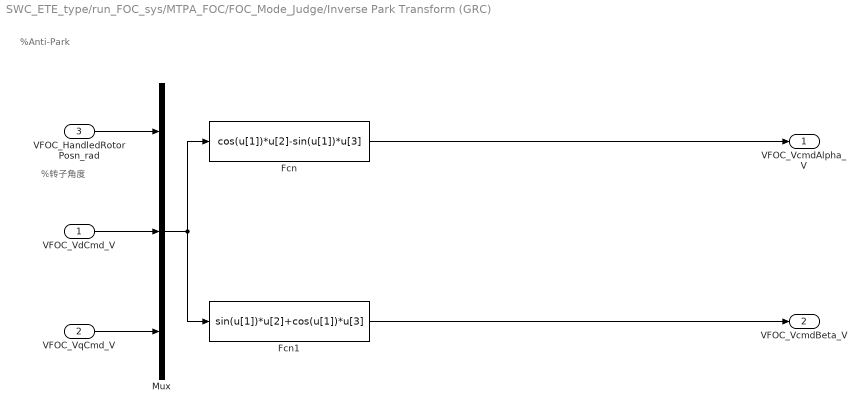
== system SWC_ETE_type/run_FOC_sys/MTPA_FOC/FOC_Mode_Judge/Inverse Park Transform (GRC) ==
  note: %转子角度
  note: %Anti-Park
  VFOC_VdCmd_V : Inport
  VFOC_VqCmd_V : Inport  Port=2
  VFOC_HandledRotorPosn_rad : Inport  Port=3
  Fcn : Fcn  Expr=cos(u[1])*u[2]-sin(u[1])*u[3]
  Fcn1 : Fcn  Expr=sin(u[1])*u[2]+cos(u[1])*u[3]
  Mux : Mux  Inputs=3
  VFOC_VcmdAlpha_V : Outport
  VFOC_VcmdBeta_V : Outport  Port=2
  wires:
  VFOC_HandledRotorPosn_rad/1 -> Mux/1
  Mux/1 -> Fcn/1, Fcn1/1
  VFOC_VdCmd_V/1 -> Mux/2
  VFOC_VqCmd_V/1 -> Mux/3
  Fcn1/1 -> VFOC_VcmdBeta_V/1
  Fcn/1 -> VFOC_VcmdAlpha_V/1

== system SWC_ETE_type/run_FOC_sys/MTPA_FOC/PWM_idle_Mode/Enabled Subsystem ==
  Enable : EnablePort  StatesWhenEnabling=reset
  C Caller1 : CCaller  FunctionName=pwm_set_idle
